simulink model "CANopen_CAN_Sender_Receiver"  (R2021b)
settings: Solver=VariableStepAuto  StartTime=0.0  StopTime=10.0  RelTol=1e-3
undefined symbols (not defined in the file): canChannel
libraries: simulink x48, commutil2 x5, canlib x3, dspindex x3, etargetslib x2, canmsglib x1
(part 1 of 2)
settings Model: Creator=adhip  LastModifiedBy=adhip

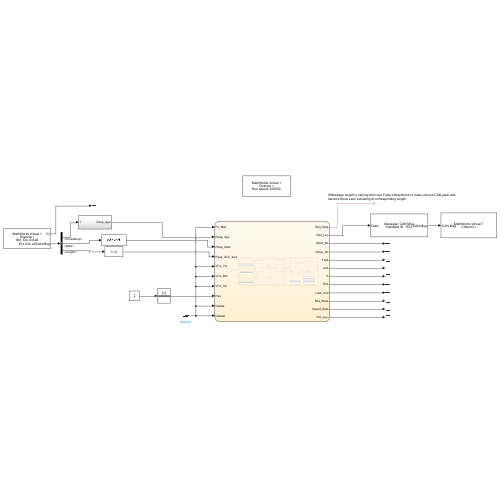
[thumbnail: Simulink's stored preview of the top-level diagram]
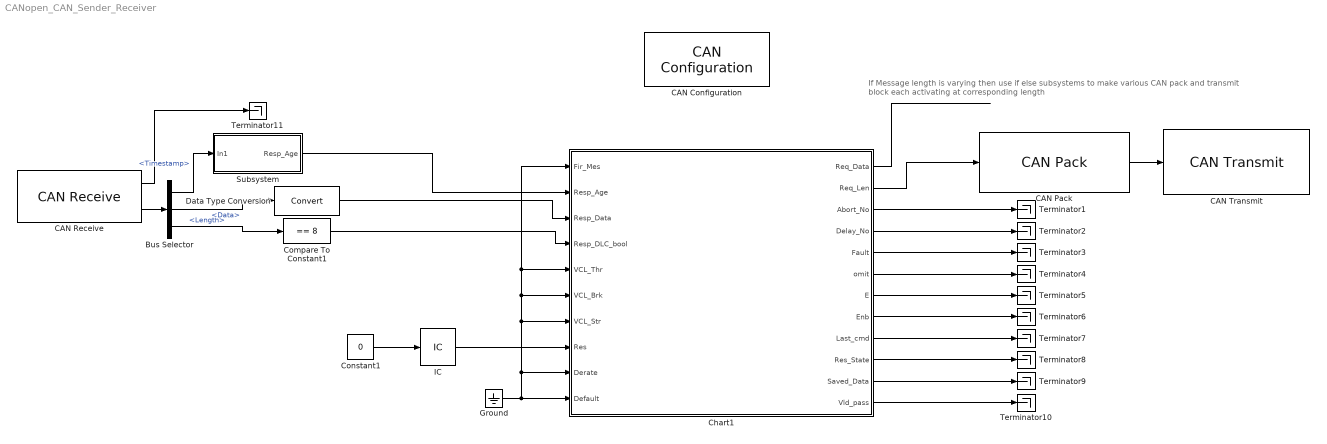
== system CANopen_CAN_Sender_Receiver ==
  note: If Message length is varying then use if else subsystems to make various CAN pack and transmit block each activating at corresponding length
  Bus Selector : BusSelector  OutputSignals=Timestamp,Data,Length
  CAN Configuration : canlib/CAN Configuration  BlockHandle=3200.0002  Device=MathWorks Virtual 1 (Channel 1)  DeviceMenu=MathWorks Virtual 1 (Channel 1)  ObjConstructor=canChannel('MathWorks', 'Virtual 1', 1)  BusSpeed=500000  EnableBitParameters=off  AckMode=Normal
      settings: SourceProductBaseCode=VN
  CAN Pack : canmsglib/CAN Pack  MsgList=(none)  MsgName=CAN Msg  MsgIDType=Standard (11-bit identifier)  MsgIdentifier=1574  MsgLength=8  Remote=off  ApplyMinMax=off  BusOutput=off  SignalInfo={}
      settings: SourceProductBaseCode=ME,XP,VN  DataFormat=raw data
  CAN Receive : canlib/CAN Receive  BlockHandle=3202.0002  Device=MathWorks Virtual 1 (Channel 1)  DeviceMenu=MathWorks Virtual 1 (Channel 1)  ObjConstructor=canChannel('MathWorks', 'Virtual 1', 1)  EnableStandardIDsFilter=off  StdIDsCombo=Allow only  StandardIDs=0x5a6  EnableExtendedIDsFilter=off  ExtIDsCombo=Allow all  ExtendedIDs=0  SampleTime=0.01  MsgsPerTimestep=all  InternalFilterUpdateStatus=on  BusOutput=on
      settings: SourceProductBaseCode=VN
  CAN Transmit : canlib/CAN Transmit  BlockHandle=3203.0002  Device=MathWorks Virtual 1 (Channel 1)  DeviceMenu=MathWorks Virtual 1 (Channel 1)  ObjConstructor=canChannel('MathWorks', 'Virtual 1', 1)  EnableEventTransmit=off  EnablePeriodicTransmit=off  MessagePeriod=1.000
      settings: SourceProductBaseCode=VN
  Chart1 : Stateflow chart  TreatAsAtomicUnit=on
      settings: PortSchema="{\"entries\":[{\"content\":{\"sides\":[{\"content\":{\"connectorIds\":[\"In10\",\"In1\",\"In3\",\"In2\",\"In4\",\"In5\",\"In6\",\"In9\",\"In7\",\"In8\"]},\"type\":\"ConnectorPlacement.EquallySpacedRectSide\",\"uuid\":\"d6208ab0-0bb6-4095-9d61-a018a45d5454\"},{\"content\":{\"connectorIds\":[\"Out1\",\"Out2\",\"Out3\",\"Out4\",\"Out5\",\"Out6\",\"Out7\",\"Out8\",\"Out9\",\"Out10\",\"Out11\",\"Out12\"],\"side\":\"RIGHT\"},\"type\":\"ConnectorPlacement.EquallySpacedRectSide\",\"uuid\":\"26e1aa46-d8b9-4154-9ae7-d888c7233d2e\"},{\"content\":{\"connectorIds\":[],\"side\":\"TOP\"},\"type\":\"ConnectorPlacement.EquallySpacedRectSide\",\"uuid\":\"42ea1899-a59d-4e0e-aa36-3438d8e67875\"}]},\"type\":\"ConnectorPlacement.EquallySpacedConnector\",\"uuid\":\"78564ca8-fcdf-4051-a3b6-ae8f3fd9c22a\"}],\"packageUris\":[\"http://schema.mathworks.com/mf0/Connector/R2020b\"],\"version\":\"1.0\"}"
  Compare To Constant1 : simulink/Logic and Bit Operations/Compare To Constant  relop===  const=8  OutDataTypeStr=boolean
  Constant1 : Constant  Value=0
  Data Type Conversion : DataTypeConversion
  Ground : Ground
  IC : InitialCondition
  Subsystem : Subsystem
  Terminator{1..11} (11 alike) : Terminator
  wires:
  Constant1/1 -> IC/1
  Ground/1 -> Chart1/8(Default), Chart1/6(VCL_Str), Chart1/5(VCL_Brk), Chart1/4(VCL_Thr), Chart1/10(Fir_Mes), Chart1/7(Derate)
  IC/1 -> Chart1/9(Res)
  CAN Receive/2 -> Bus Selector/1
  Bus Selector/3 -> Compare To Constant1/1  "<Length>"
  Compare To Constant1/1 -> Chart1/2(Resp_DLC_bool)
  Bus Selector/2 -> Data Type Conversion/1  "<Data>"
  Data Type Conversion/1 -> Chart1/3(Resp_Data)
  Bus Selector/1 -> Subsystem/1(In1)  "<Timestamp>"
  Subsystem/1(Resp_Age) -> Chart1/1(Resp_Age)
  Chart1/6(omit) -> Terminator4/1
  Chart1/11(Saved_Data) -> Terminator9/1
  Chart1/10(Res_State) -> Terminator8/1
  Chart1/7(E) -> Terminator5/1
  Chart1/9(Last_cmd) -> Terminator7/1
  Chart1/5(Fault) -> Terminator3/1
  Chart1/4(Delay_No) -> Terminator2/1
  Chart1/8(Enb) -> Terminator6/1
  Chart1/12(Vld_pass) -> Terminator10/1
  Chart1/3(Abort_No) -> Terminator1/1
  Chart1/1(Req_Data) -> ?
  CAN Pack/1 -> CAN Transmit/1
  Chart1/2(Req_Len) -> CAN Pack/1
  CAN Receive/1 -> Terminator11/1

== system CANopen_CAN_Sender_Receiver/Chart1/Transreceive.Identifying_Message.Disintegrate ==
  Data : Inport  OutDataTypeStr=uint8  PortDimensions=8
  f : TriggerPort  TriggerType=function-call  VariantControl=(inherit)
      settings: CopyFcn=Stateflow.SLINSF.SimulinkMan.removeBlockPreDeleteFcn  PreDeleteFcn=Stateflow.SLINSF.SimulinkMan.unsafePredeleteFcn
  Expedite : Subsystem
  Gains : Subsystem
  NOT : Logic  Operator=NOT  IconShape=distinctive  AllPortsSameDT=off  OutDataTypeStr=boolean
  Segmented : Subsystem  TreatAsAtomicUnit=on
  Subsystem : Subsystem
  Switch1 : Switch  Criteria=u2 > Threshold
  Switch2 : Switch  Criteria=u2 > Threshold
  Terminator : Terminator
  Terminator1 : Terminator
  Unit Delay : UnitDelay  SampleTime=-1  HasFrameUpgradeWarning=on
  Mes_No : Outport  OutDataTypeStr=uint8
  Act_Data : Outport  Port=2
  Seg_Req : Outport  Port=3  OutDataTypeStr=boolean
  Abort : Outport  Port=4  OutDataTypeStr=uint8
  wires:
  Switch1/1 -> Gains/2(Data)
  Data/1 -> Expedite/1(Data), Segmented/1(Data)
  Expedite/4("Request for Segmented Read ") -> Subsystem/1(set)
  Subsystem/1(Current State) -> Seg_Req/1, Unit Delay/1
  Segmented/1(Reset) -> Subsystem/2(Reset)
  NOT/1 -> Expedite/Enable, Switch2/2, Switch1/2
  Expedite/3(Act_Data) -> Switch1/1
  Expedite/2(Expedite) -> Terminator/1
  Segmented/2(Act_Data) -> Switch1/3
  Expedite/1(Msg No) -> Gains/1(Msg No), Mes_No/1
  Unit Delay/1 -> Segmented/Enable, NOT/1
  Expedite/5(Abort) -> Switch2/1
  Switch2/1 -> Abort/1
  Gains/1(Engineering value) -> Act_Data/1
  Segmented/4(Toggle) -> Terminator1/1
  Segmented/3(Abort) -> Switch2/3

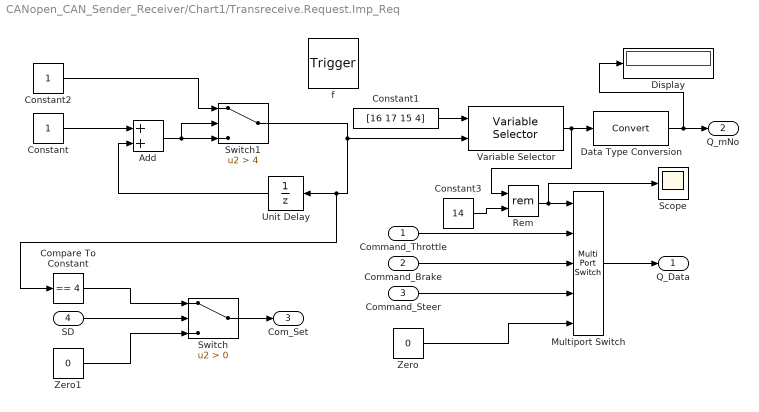
== system CANopen_CAN_Sender_Receiver/Chart1/Transreceive.Request.Imp_Req ==
  Command_Throttle : Inport  OutDataTypeStr=int8  PortDimensions=1
  Command_Brake : Inport  Port=2  OutDataTypeStr=int8  PortDimensions=1
  Command_Steer : Inport  Port=3  OutDataTypeStr=int8  PortDimensions=1
  SD : Inport  Port=4  OutDataTypeStr=boolean  PortDimensions=1
  f : TriggerPort  TriggerType=function-call  VariantControl=(inherit)
      settings: CopyFcn=Stateflow.SLINSF.SimulinkMan.removeBlockPreDeleteFcn  PreDeleteFcn=Stateflow.SLINSF.SimulinkMan.unsafePredeleteFcn
  Add : Sum
  Compare To Constant : simulink/Logic and Bit Operations/Compare To Constant  relop===  const=4  OutDataTypeStr=boolean
  Constant : Constant
  Constant1 : Constant  Value=[16 17 15 4]
  Constant2 : Constant
  Constant3 : Constant  Value=14
  Data Type Conversion : DataTypeConversion
  Display : Display
  Multiport Switch : MultiPortSwitch  Inputs=4  DiagnosticForDefault=None
  Rem : Math  Operator=rem  SaturateOnIntegerOverflow=on
  Scope : Scope
  Switch : Switch  Criteria=u2 > Threshold
  Switch1 : Switch  Criteria=u2 > Threshold  Threshold=4
  Unit Delay : UnitDelay  SampleTime=-1  HasFrameUpgradeWarning=on
  Variable Selector : dspindex/Variable Selector  NumInputs=1  rowsOrCols=Rows  IdxMode=Variable  Elements=[1 3]  ZerOneIdxMode=One-based  errmode=Clip Index  FillMode=on  FillValues=0
  Zero : Constant  Value=0  OutDataTypeStr=Inherit: Inherit via back propagation
  Zero1 : Constant  Value=0  OutDataTypeStr=Inherit: Inherit via back propagation
  Q_Data : Outport  OutDataTypeStr=uint16
  Q_mNo : Outport  Port=2  OutDataTypeStr=uint8
  Com_Set : Outport  Port=3
  wires:
  Unit Delay/1 -> Add/2
  Add/1 -> Switch1/2, Switch1/3
  Multiport Switch/1 -> Q_Data/1
  Command_Steer/1 -> Multiport Switch/4
  Command_Brake/1 -> Multiport Switch/3
  Command_Throttle/1 -> Multiport Switch/2
  Constant3/1 -> Rem/2
  Constant1/1 -> Variable Selector/1
  Constant/1 -> Add/1
  Variable Selector/1 -> Rem/1, Data Type Conversion/1
  Constant2/1 -> Switch1/1
  Zero/1 -> Multiport Switch/5
  Switch1/1 -> Compare To Constant/1, Unit Delay/1, Variable Selector/2
  Rem/1 -> Scope/1, Multiport Switch/1
  Compare To Constant/1 -> Switch/1
  Switch/1 -> Com_Set/1
  SD/1 -> Switch/2
  Zero1/1 -> Switch/3
  Data Type Conversion/1 -> Q_mNo/1, Display/1

== system CANopen_CAN_Sender_Receiver/Chart1/Transreceive.Request.Logic_Based ==
  f : TriggerPort  TriggerType=function-call  VariantControl=(inherit)
      settings: CopyFcn=Stateflow.SLINSF.SimulinkMan.removeBlockPreDeleteFcn  PreDeleteFcn=Stateflow.SLINSF.SimulinkMan.unsafePredeleteFcn
  Add : Sum
  Constant : Constant
  Constant1 : Constant  Value=[12 13 10 11]
  Constant2 : Constant
  Data Type Conversion : DataTypeConversion
  Display : Display
  Switch1 : Switch  Criteria=u2 > Threshold  Threshold=4
  Unit Delay : UnitDelay  SampleTime=-1  HasFrameUpgradeWarning=on
  Variable Selector : dspindex/Variable Selector  NumInputs=1  rowsOrCols=Rows  IdxMode=Variable  Elements=[1 3]  ZerOneIdxMode=One-based  errmode=Clip Index  FillMode=on  FillValues=0
  Zero : Constant  Value=0  OutDataTypeStr=Inherit: Inherit via back propagation
  Zero1 : Constant  Value=0  OutDataTypeStr=Inherit: Inherit via back propagation
  Q_Data : Outport  OutDataTypeStr=uint16
  Q_mNo : Outport  Port=2  OutDataTypeStr=uint8
  Com_Set : Outport  Port=3
  wires:
  Unit Delay/1 -> Add/2
  Add/1 -> Switch1/2, Switch1/3
  Constant1/1 -> Variable Selector/1
  Constant/1 -> Add/1
  Variable Selector/1 -> Data Type Conversion/1
  Constant2/1 -> Switch1/1
  Zero/1 -> Q_Data/1
  Switch1/1 -> Variable Selector/2, Unit Delay/1
  Zero1/1 -> Com_Set/1
  Data Type Conversion/1 -> Q_mNo/1, Display/1

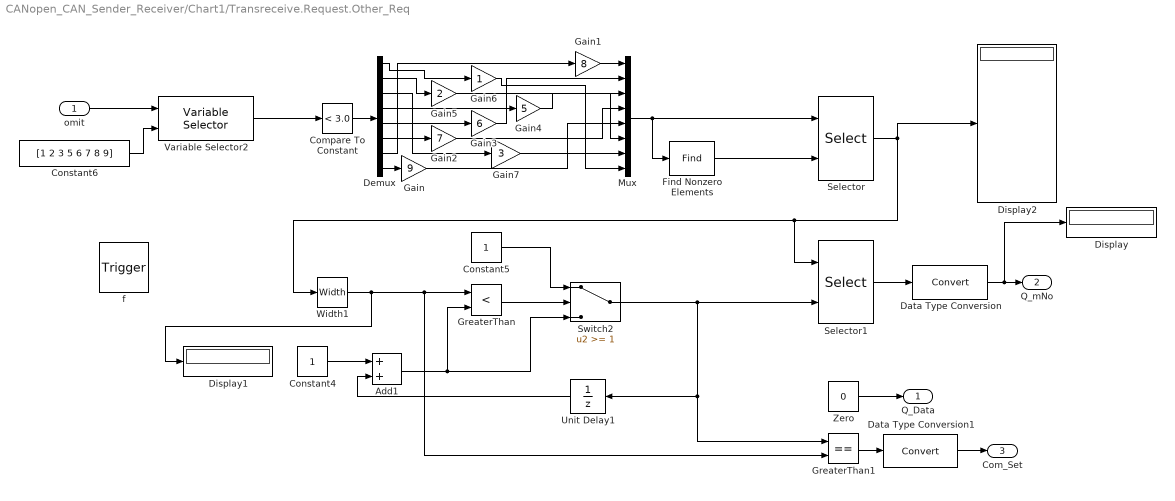
== system CANopen_CAN_Sender_Receiver/Chart1/Transreceive.Request.Other_Req ==
  omit : Inport  OutDataTypeStr=uint8  PortDimensions=17
  f : TriggerPort  TriggerType=function-call  VariantControl=(inherit)
      settings: CopyFcn=Stateflow.SLINSF.SimulinkMan.removeBlockPreDeleteFcn  PreDeleteFcn=Stateflow.SLINSF.SimulinkMan.unsafePredeleteFcn
  Add1 : Sum
  Compare To Constant : simulink/Logic and Bit Operations/Compare To Constant  relop=<  const=3.0  OutDataTypeStr=boolean
  Constant4 : Constant
  Constant5 : Constant
  Constant6 : Constant  Value=[1 2 3 5 6 7 8 9]
  Data Type Conversion : DataTypeConversion
  Data Type Conversion1 : DataTypeConversion
  Demux : Demux  Outputs=8
  Display : Display
  Display1 : Display
  Display2 : Display
  Find Nonzero Elements : Find  NumberOfInputDimensions=3
  Gain : Gain  Gain=9  OutDataTypeStr=uint8
  Gain1 : Gain  Gain=8  OutDataTypeStr=uint8
  Gain2 : Gain  Gain=7  OutDataTypeStr=uint8
  Gain3 : Gain  Gain=6  OutDataTypeStr=uint8
  Gain4 : Gain  Gain=5  OutDataTypeStr=uint8
  Gain5 : Gain  Gain=2  OutDataTypeStr=uint8
  Gain6 : Gain  OutDataTypeStr=uint8
  Gain7 : Gain  Gain=3  OutDataTypeStr=uint8
  GreaterThan : RelationalOperator  Operator=<  OutDataTypeStr=boolean  RndMeth=Simplest
  GreaterThan1 : RelationalOperator  Operator===  OutDataTypeStr=boolean  RndMeth=Simplest
  Mux : Mux  Inputs=8
  Selector : Selector  InputPortWidth=8  IndexOptions=Index vector (port)  Indices=[1 3]  OutputSizes=1
  Selector1 : Selector  InputPortWidth=8  IndexOptions=Index vector (port)  Indices=[1 3]  OutputSizes=1
  Switch2 : Switch  Threshold=1
  Unit Delay1 : UnitDelay  SampleTime=-1  HasFrameUpgradeWarning=on
  Variable Selector2 : dspindex/Variable Selector  NumInputs=1  rowsOrCols=Rows  IdxMode=Variable  Elements=[1 3]  ZerOneIdxMode=One-based  errmode=Clip Index  FillMode=on  FillValues=0
  Width1 : Width
  Zero : Constant  Value=0  OutDataTypeStr=Inherit: Inherit via back propagation
  Q_Data : Outport  OutDataTypeStr=uint16
  Q_mNo : Outport  Port=2  OutDataTypeStr=uint8
  Com_Set : Outport  Port=3
  wires:
  Zero/1 -> Q_Data/1
  Switch2/1 -> Selector1/2, GreaterThan1/1, Unit Delay1/1
  Gain/1 -> Mux/5
  Gain6/1 -> Mux/8
  Demux/7 -> Gain1/1
  Demux/1 -> Gain6/1
  Gain3/1 -> Mux/2
  Gain5/1 -> Mux/6
  Demux/3 -> Gain7/1
  Demux/4 -> Gain4/1
  Demux/2 -> Gain5/1
  Mux/1 -> Selector/1, Find Nonzero Elements/1
  Demux/8 -> Gain/1
  Width1/1 -> GreaterThan1/2, GreaterThan/1, Display1/1
  Constant6/1 -> Variable Selector2/2
  Compare To Constant/1 -> Demux/1
  Demux/6 -> Gain2/1
  Constant5/1 -> Switch2/1
  Unit Delay1/1 -> Add1/2
  Demux/5 -> Gain3/1
  Gain4/1 -> Mux/3
  Constant4/1 -> Add1/1
  Add1/1 -> GreaterThan/2, Switch2/3
  Gain2/1 -> Mux/4
  Selector1/1 -> Data Type Conversion/1
  Selector/1 -> Selector1/1, Width1/1, Display2/1
  Variable Selector2/1 -> Compare To Constant/1
  GreaterThan/1 -> Switch2/2
  omit/1 -> Variable Selector2/1
  Gain7/1 -> Mux/7
  Find Nonzero Elements/1 -> Selector/2
  Gain1/1 -> Mux/1
  GreaterThan1/1 -> Data Type Conversion1/1
  Data Type Conversion/1 -> Q_mNo/1, Display/1
  Data Type Conversion1/1 -> Com_Set/1

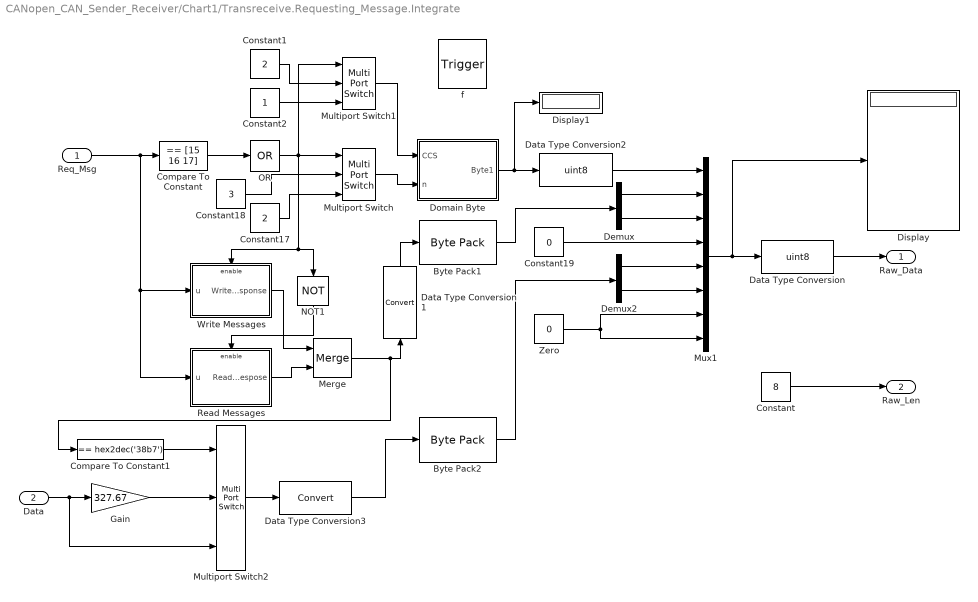
== system CANopen_CAN_Sender_Receiver/Chart1/Transreceive.Requesting_Message.Integrate ==
  Req_Msg : Inport  OutDataTypeStr=uint8  PortDimensions=1
  Data : Inport  Port=2  OutDataTypeStr=uint16  PortDimensions=1
  f : TriggerPort  TriggerType=function-call  VariantControl=(inherit)
      settings: CopyFcn=Stateflow.SLINSF.SimulinkMan.removeBlockPreDeleteFcn  PreDeleteFcn=Stateflow.SLINSF.SimulinkMan.unsafePredeleteFcn
  Byte Pack1 : etargetslib/Byte Pack  datatypes={'uint16'}  byteAlign=1
  Byte Pack2 : etargetslib/Byte Pack  datatypes={'uint16'}  byteAlign=1
  Compare To Constant : simulink/Logic and Bit Operations/Compare To Constant  relop===  const=[15 16 17]  OutDataTypeStr=boolean
  Compare To Constant1 : simulink/Logic and Bit Operations/Compare To Constant  relop===  const=hex2dec('38b7')  OutDataTypeStr=boolean
  Constant : Constant  Value=8  OutDataTypeStr=uint8
  Constant1 : Constant  Value=2
  Constant17 : Constant  Value=2
  Constant18 : Constant  Value=3
  Constant19 : Constant  Value=0  OutDataTypeStr=uint8
  Constant2 : Constant
  Data Type Conversion : DataTypeConversion  OutDataTypeStr=uint8
  Data Type Conversion1 : DataTypeConversion
  Data Type Conversion2 : DataTypeConversion  OutDataTypeStr=uint8
  Data Type Conversion3 : DataTypeConversion
  Demux : Demux  Outputs=2
  Demux2 : Demux  Outputs=2
  Display : Display
  Display1 : Display
  Domain Byte : Subsystem
  Gain : Gain  Gain=327.67
  Merge : Merge
  Multiport Switch : MultiPortSwitch  DataPortOrder=Zero-based contiguous  Inputs=2  zeroidx=on
  Multiport Switch1 : MultiPortSwitch  DataPortOrder=Zero-based contiguous  Inputs=2  zeroidx=on
  Multiport Switch2 : MultiPortSwitch  DataPortOrder=Zero-based contiguous  Inputs=2  zeroidx=on
  Mux1 : Mux  Inputs=8
  NOT1 : Logic  Operator=NOT  IconShape=distinctive  AllPortsSameDT=off  OutDataTypeStr=boolean
  OR : Logic  Operator=OR  Inputs=1  IconShape=distinctive  AllPortsSameDT=off  OutDataTypeStr=boolean
  Read Messages : Subsystem
  Write Messages : Subsystem
  Zero : Constant  Value=0  OutDataTypeStr=uint8
  Raw_Data : Outport
  Raw_Len : Outport  Port=2
  wires:
  Gain/1 -> Multiport Switch2/2
  Compare To Constant1/1 -> Multiport Switch2/1
  Data Type Conversion3/1 -> Byte Pack2/1
  Multiport Switch2/1 -> Data Type Conversion3/1
  Multiport Switch1/1 -> Domain Byte/1(CCS)
  Constant2/1 -> Multiport Switch1/3
  Constant1/1 -> Multiport Switch1/2
  Data Type Conversion1/1 -> Byte Pack1/1
  Demux/1 -> Mux1/2
  Data Type Conversion2/1 -> Mux1/1
  Demux2/1 -> Mux1/5
  Demux/2 -> Mux1/3
  Data/1 -> Gain/1, Multiport Switch2/3
  Byte Pack1/1 -> Demux/1
  Byte Pack2/1 -> Demux2/1
  Domain Byte/1(Byte1) -> Data Type Conversion2/1, Display1/1
  Constant19/1 -> Mux1/4
  NOT1/1 -> Read Messages/Enable
  Read Messages/1(Read_Respose) -> Merge/2
  Mux1/1 -> Data Type Conversion/1, Display/1
  Zero/1 -> Mux1/8, Mux1/7
  OR/1 -> Write Messages/Enable, NOT1/1, Multiport Switch/1, Multiport Switch1/1
  Constant18/1 -> Multiport Switch/2
  Compare To Constant/1 -> OR/1
  Demux2/2 -> Mux1/6
  Req_Msg/1 -> Read Messages/1(u), Write Messages/1(u), Compare To Constant/1
  Constant17/1 -> Multiport Switch/3
  Data Type Conversion/1 -> Raw_Data/1
  Write Messages/1(Write_response) -> Merge/1
  Merge/1 -> Data Type Conversion1/1, Compare To Constant1/1
  Multiport Switch/1 -> Domain Byte/2(n)
  Constant/1 -> Raw_Len/1

== system CANopen_CAN_Sender_Receiver/Subsystem ==
  note: Create a system that comapres time stamp with atcual time and gives age 0 if a fresh message is received
  In1 : Inport
  Clock : Clock
  Resp_Age : Outport

== system CANopen_CAN_Sender_Receiver/Chart1/Transreceive.Identifying_Message.Disintegrate/Expedite ==
  Data : Inport
  Enable : EnablePort
  Data Processing : Subsystem
  Demux : Demux  Outputs=8
  Display{,1..3} (4 alike) : Display
  MessageNumber : Subsystem
  Mux : Mux  Inputs=3
  Mux1 : Mux
  Msg No : Outport
  Expedite : Outport  Port=2
  Act_Data : Outport  Port=3
  "Request for Segmented Read " : Outport  Port=4
  Abort : Outport  Port=5
  wires:
  Demux/8 -> Mux1/4
  Demux/3 -> Mux/2
  Demux/5 -> Mux1/1
  Demux/7 -> Mux1/3
  Mux/1 -> MessageNumber/2(u)
  Demux/4 -> Mux/3
  Demux/2 -> Mux/1
  Mux1/1 -> Data Processing/2(In1), Display/1
  Demux/6 -> Mux1/2
  Demux/1 -> MessageNumber/1(Domain Info)
  MessageNumber/1(Msg No) -> Data Processing/1(Msg No), Msg No/1, Display1/1
  MessageNumber/2(Expedite) -> Expedite/1
  Data/1 -> Demux/1, Display2/1
  MessageNumber/3("Request for Segmented Read ") -> "Request for Segmented Read "/1
  Data Processing/1(Act_Data) -> Act_Data/1, Display3/1
  MessageNumber/4(Abort) -> Abort/1

== system CANopen_CAN_Sender_Receiver/Chart1/Transreceive.Identifying_Message.Disintegrate/Gains ==
  Msg No : Inport
  Data : Inport  Port=2
  Constant : Constant  Value=[327.67, 327.67, 1, 1, 10, 10, 10, 1, 1, 40.96, 40.96, 40.96, 40.96, 105, 1, 1, 1, 1]
  Demux : Demux  Outputs=18
  Display : Display
  Display1 : Display
  Divide : Product  Inputs=*/
  Multiport Switch : MultiPortSwitch  Inputs=18
  Engineering value : Outport
  wires:
  Multiport Switch/1 -> Divide/2, Display/1
  Data/1 -> Divide/1
  Divide/1 -> Engineering value/1, Display1/1
  Msg No/1 -> Multiport Switch/1
  Demux/1 -> Multiport Switch/2
  Demux/2 -> Multiport Switch/3
  Demux/3 -> Multiport Switch/4
  Demux/4 -> Multiport Switch/5
  Demux/5 -> Multiport Switch/6
  Demux/6 -> Multiport Switch/7
  Demux/7 -> Multiport Switch/8
  Demux/8 -> Multiport Switch/9
  Demux/9 -> Multiport Switch/10
  Demux/10 -> Multiport Switch/11
  Demux/11 -> Multiport Switch/12
  Demux/12 -> Multiport Switch/13
  Demux/13 -> Multiport Switch/14
  Demux/14 -> Multiport Switch/15
  Demux/15 -> Multiport Switch/16
  Demux/16 -> Multiport Switch/17
  Demux/17 -> Multiport Switch/18
  Demux/18 -> Multiport Switch/19
  Constant/1 -> Demux/1

== system CANopen_CAN_Sender_Receiver/Chart1/Transreceive.Identifying_Message.Disintegrate/Segmented ==
  Data : Inport
  Enable : EnablePort
  Data Processing : Subsystem
  Demux : Demux  Outputs=8
  MessageNumber : Subsystem
  Mux1 : Mux  Inputs=7
  Terminator : Terminator
  Terminator1 : Terminator
  Reset : Outport
  Act_Data : Outport  Port=2
  Abort : Outport  Port=3
  Toggle : Outport  Port=4
  wires:
  Demux/1 -> MessageNumber/1(Domain Info)
  Data/1 -> Demux/1
  Mux1/1 -> Data Processing/1(Data)
  Demux/2 -> Mux1/1
  Demux/4 -> Mux1/3
  Demux/3 -> Mux1/2
  MessageNumber/2(Reset) -> Reset/1
  Demux/5 -> Mux1/4
  Demux/6 -> Mux1/5
  Demux/7 -> Mux1/6
  Demux/8 -> Mux1/7
  Data Processing/1(Act_Data) -> Act_Data/1
  MessageNumber/1(Abort) -> Abort/1
  MessageNumber/3(Toggle) -> Toggle/1
  MessageNumber/5(Segmented Response) -> Terminator/1
  MessageNumber/4(Error SCS) -> Terminator1/1

== system CANopen_CAN_Sender_Receiver/Chart1/Transreceive.Identifying_Message.Disintegrate/Subsystem ==
  set : Inport
  Reset : Inport  Port=2
  Constant : Constant  Value=0  OutDataTypeStr=boolean
  Constant1 : Constant  OutDataTypeStr=boolean
  Multiport Switch : MultiPortSwitch  DataPortOrder=Zero-based contiguous  Inputs=2  zeroidx=on
  Multiport Switch1 : MultiPortSwitch  DataPortOrder=Zero-based contiguous  Inputs=2  zeroidx=on
  Unit Delay : UnitDelay  SampleTime=-1  HasFrameUpgradeWarning=on
  Current State : Outport
  wires:
  Multiport Switch/1 -> Current State/1, Unit Delay/1
  Constant/1 -> Multiport Switch/3
  Multiport Switch1/1 -> Multiport Switch/2
  Constant1/1 -> Multiport Switch1/3
  Unit Delay/1 -> Multiport Switch1/2
  Reset/1 -> Multiport Switch/1
  set/1 -> Multiport Switch1/1

== system CANopen_CAN_Sender_Receiver/Chart1/Transreceive.Requesting_Message.Integrate/Domain Byte ==
  CCS : Inport
  n : Inport  Port=2
  Bit to Integer Converter : commutil2/Bit to Integer Converter  nbits=8  bitOrder=MSB first  signedOutputValues=Unsigned  outDtype=Inherit via internal rule  outDtypeSigned=Inherit via internal rule
      settings: SourceProductBaseCode=SL
  Constant : Constant  Value=0
  Constant1 : Constant  Value=0
  Constant2 : Constant
  Constant3 : Constant  Value=0
  Constant4 : Constant
  Constant5 : Constant
  Demux : Demux  Outputs=2
  Demux1 : Demux  Outputs=2
  Display1 : Display
  Display2 : Display
  Integer to Bit Converter : commutil2/Integer to Bit Converter  nbits=2  signedInputValues=Unsigned  bitOrder=MSB first  outDtype=Inherit via internal rule
      settings: SourceProductBaseCode=SL
  Integer to Bit Converter1 : commutil2/Integer to Bit Converter  nbits=2  signedInputValues=Unsigned  bitOrder=MSB first  outDtype=Inherit via internal rule
      settings: SourceProductBaseCode=SL
  Mux : Mux  Inputs=8
  Byte1 : Outport
  wires:
  CCS/1 -> Integer to Bit Converter1/1
  Integer to Bit Converter1/1 -> Demux1/1, Display2/1
  Mux/1 -> Bit to Integer Converter/1, Display1/1
  Bit to Integer Converter/1 -> Byte1/1
  Demux1/1 -> Mux/2
  Demux1/2 -> Mux/3
  Constant4/1 -> Mux/8
  Constant/1 -> Mux/1
  Constant3/1 -> Mux/4
  Constant5/1 -> Mux/7
  n/1 -> Integer to Bit Converter/1
  Integer to Bit Converter/1 -> Demux/1
  Demux/1 -> Mux/5
  Demux/2 -> Mux/6

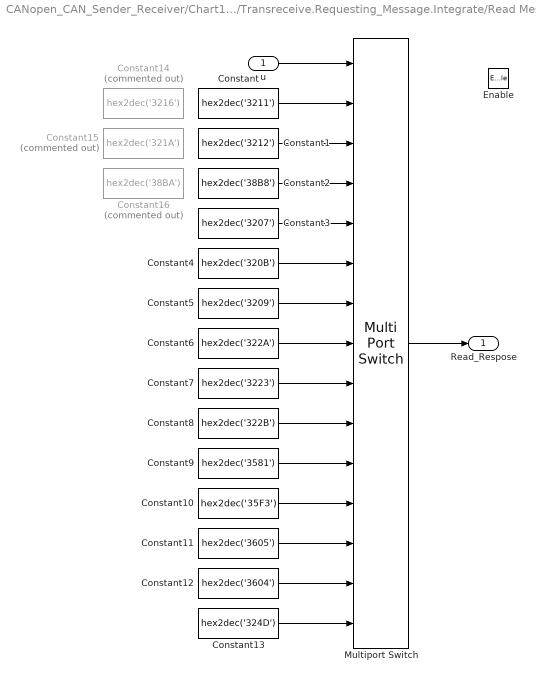
== system CANopen_CAN_Sender_Receiver/Chart1/Transreceive.Requesting_Message.Integrate/Read Messages ==
  u : Inport
  Enable : EnablePort  StatesWhenEnabling=reset
  Constant : Constant  Value=hex2dec('3211')
  Constant1 : Constant  Value=hex2dec('3212')
  Constant10 : Constant  Value=hex2dec('35F3')
  Constant11 : Constant  Value=hex2dec('3605')
  Constant12 : Constant  Value=hex2dec('3604')
  Constant13 : Constant  Value=hex2dec('324D')
  Constant14 : Constant  Commented=on  Value=hex2dec('3216')
  Constant15 : Constant  Commented=on  Value=hex2dec('321A')
  Constant16 : Constant  Commented=on  Value=hex2dec('38BA')
  Constant2 : Constant  Value=hex2dec('38B8')
  Constant3 : Constant  Value=hex2dec('3207')
  Constant4 : Constant  Value=hex2dec('320B')
  Constant5 : Constant  Value=hex2dec('3209')
  Constant6 : Constant  Value=hex2dec('322A')
  Constant7 : Constant  Value=hex2dec('3223')
  Constant8 : Constant  Value=hex2dec('322B')
  Constant9 : Constant  Value=hex2dec('3581')
  Multiport Switch : MultiPortSwitch  Inputs=14
  Read_Respose : Outport
  wires:
  u/1 -> Multiport Switch/1
  Constant/1 -> Multiport Switch/2
  Constant1/1 -> Multiport Switch/3
  Constant3/1 -> Multiport Switch/5
  Constant2/1 -> Multiport Switch/4
  Constant7/1 -> Multiport Switch/9
  Constant6/1 -> Multiport Switch/8
  Constant5/1 -> Multiport Switch/7
  Constant4/1 -> Multiport Switch/6
  Constant8/1 -> Multiport Switch/10
  Constant9/1 -> Multiport Switch/11
  Constant10/1 -> Multiport Switch/12
  Constant11/1 -> Multiport Switch/13
  Constant12/1 -> Multiport Switch/14
  Constant13/1 -> Multiport Switch/15
  Multiport Switch/1 -> Read_Respose/1

== system CANopen_CAN_Sender_Receiver/Chart1/Transreceive.Requesting_Message.Integrate/Write Messages ==
  u : Inport
  Enable : EnablePort  StatesWhenEnabling=reset
  Add : Sum  Inputs=+++
  Constant : Constant  Value=hex2dec('3218')
  Constant1 : Constant  Value=hex2dec('3219')
  Constant2 : Constant  Value=hex2dec('38b7')
  Gain1 : Gain  Gain=2  OutDataTypeStr=uint16
  Gain3 : Gain  Gain=3  OutDataTypeStr=uint16
  Multiport Switch : MultiPortSwitch
  VCL_Brake : simulink/Logic and Bit Operations/Compare To Constant  relop===  const=16  OutDataTypeStr=uint8
  VCL_Steer : simulink/Logic and Bit Operations/Compare To Constant  relop===  const=17  OutDataTypeStr=uint8
  VCL_Throttle : simulink/Logic and Bit Operations/Compare To Constant  relop===  const=15  OutDataTypeStr=uint8
  Write_response : Outport
  wires:
  VCL_Brake/1 -> Gain1/1
  u/1 -> VCL_Steer/1, VCL_Brake/1, VCL_Throttle/1
  VCL_Steer/1 -> Gain3/1
  Multiport Switch/1 -> Write_response/1
  Gain1/1 -> Add/2
  VCL_Throttle/1 -> Add/1
  Gain3/1 -> Add/3
  Add/1 -> Multiport Switch/1
  Constant/1 -> Multiport Switch/2
  Constant2/1 -> Multiport Switch/4
  Constant1/1 -> Multiport Switch/3

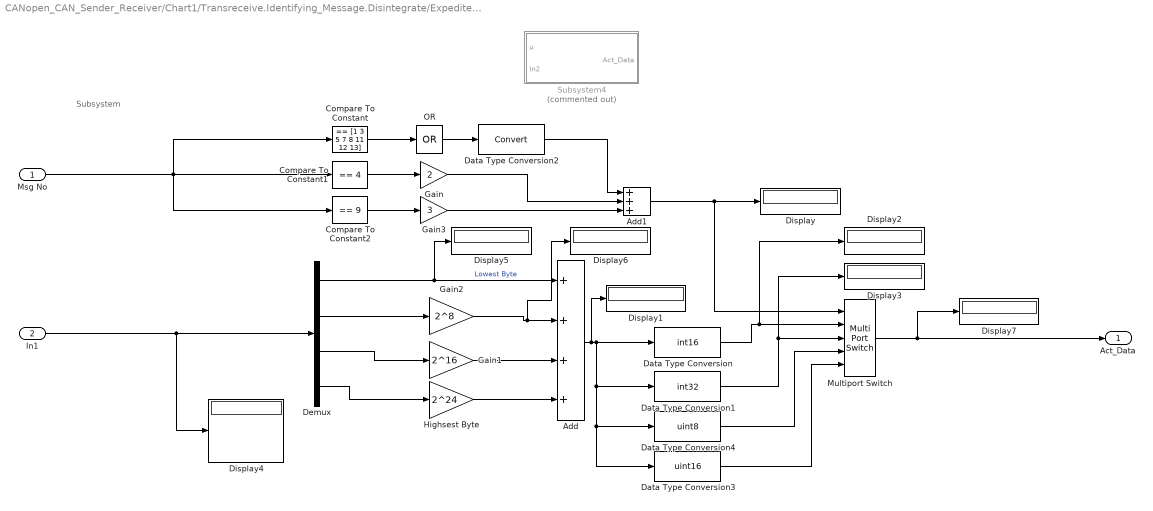
== system CANopen_CAN_Sender_Receiver/Chart1/Transreceive.Identifying_Message.Disintegrate/Expedite/Data Processing ==
  note: Subsystem
  Msg No : Inport
  In1 : Inport  Port=2
  Add : Sum  Inputs=++++  OutDataTypeStr=uint32
  Add1 : Sum  Inputs=+++
  Compare To Constant : simulink/Logic and Bit Operations/Compare To Constant  relop===  const=[1 3 5 7 8 11 12 13]  OutDataTypeStr=boolean
  Compare To Constant1 : simulink/Logic and Bit Operations/Compare To Constant  relop===  const=4  OutDataTypeStr=boolean
  Compare To Constant2 : simulink/Logic and Bit Operations/Compare To Constant  relop===  const=9  OutDataTypeStr=boolean
  Data Type Conversion : DataTypeConversion  OutDataTypeStr=int16  SaturateOnIntegerOverflow=on
  Data Type Conversion1 : DataTypeConversion  OutDataTypeStr=int32  SaturateOnIntegerOverflow=on
  Data Type Conversion2 : DataTypeConversion
  Data Type Conversion3 : DataTypeConversion  OutDataTypeStr=uint16  SaturateOnIntegerOverflow=on
  Data Type Conversion4 : DataTypeConversion  OutDataTypeStr=uint8  SaturateOnIntegerOverflow=on
  Demux : Demux
  Display{,1..7} (8 alike) : Display
  Gain : Gain  Gain=2
  Gain1 : Gain  Gain=2^16
  Gain2 : Gain  Gain=2^8
  Gain3 : Gain  Gain=3
  Highsest Byte : Gain  Gain=2^24
  Multiport Switch : MultiPortSwitch  Inputs=4  DiagnosticForDefault=None  OutDataTypeStr=double
  OR : Logic  Operator=OR  Inputs=1  IconShape=distinctive  AllPortsSameDT=off  OutDataTypeStr=boolean
  Subsystem4 : Subsystem  Commented=on
  Act_Data : Outport
  wires:
  Gain/1 -> Add1/2
  In1/1 -> Display4/1, Demux/1
  Demux/4 -> Highsest Byte/1
  Add1/1 -> Multiport Switch/1, Display/1
  Data Type Conversion4/1 -> Multiport Switch/4
  Data Type Conversion1/1 -> Multiport Switch/3, Display3/1
  Data Type Conversion2/1 -> Add1/1
  Compare To Constant/1 -> OR/1
  Compare To Constant2/1 -> Gain3/1
  Gain3/1 -> Add1/3
  Highsest Byte/1 -> Add/4
  OR/1 -> Data Type Conversion2/1
  Demux/1 -> Display5/1, Add/1  "Lowest Byte"
  Data Type Conversion3/1 -> Multiport Switch/5
  Gain2/1 -> Display6/1, Add/2
  Gain1/1 -> Add/3
  Data Type Conversion/1 -> Multiport Switch/2, Display2/1
  Compare To Constant1/1 -> Gain/1
  Demux/2 -> Gain2/1
  Demux/3 -> Gain1/1
  Msg No/1 -> Compare To Constant/1, Compare To Constant1/1, Compare To Constant2/1
  Add/1 -> Display1/1, Data Type Conversion/1, Data Type Conversion1/1, Data Type Conversion4/1, Data Type Conversion3/1
  Multiport Switch/1 -> Display7/1, Act_Data/1

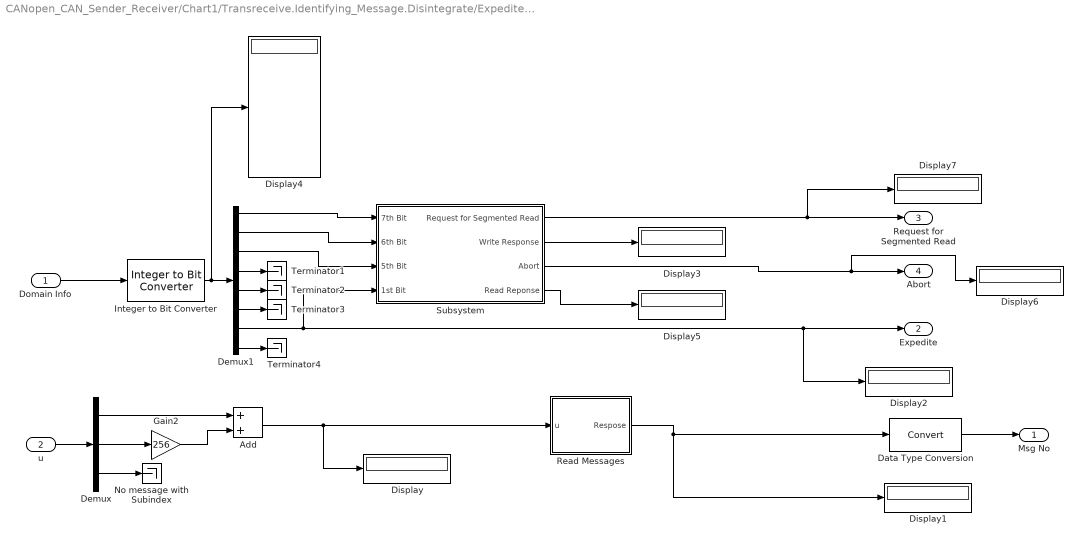
== system CANopen_CAN_Sender_Receiver/Chart1/Transreceive.Identifying_Message.Disintegrate/Expedite/MessageNumber ==
  Domain Info : Inport
  u : Inport  Port=2
  Add : Sum  OutDataTypeStr=uint16
  Data Type Conversion : DataTypeConversion
  Demux : Demux  Outputs=3
  Demux1 : Demux  Outputs=8
  Display{,1..7} (8 alike) : Display
  Gain2 : Gain  Gain=256
  Integer to Bit Converter : commutil2/Integer to Bit Converter  nbits=8  signedInputValues=Unsigned  bitOrder=MSB first  outDtype=Inherit via internal rule
      settings: SourceProductBaseCode=SL
  No message with Subindex : Terminator
  Read Messages : Subsystem
  Subsystem : Subsystem
  Terminator{1..4} (4 alike) : Terminator
  Msg No : Outport
  Expedite : Outport  Port=2
  "Request for Segmented Read " : Outport  Port=3
  Abort : Outport  Port=4
  wires:
  Subsystem/2(Write Response) -> Display3/1
  Data Type Conversion/1 -> Msg No/1
  Read Messages/1(Respose) -> Display1/1, Data Type Conversion/1
  u/1 -> Demux/1
  Demux/2 -> Gain2/1
  Demux/1 -> Add/1
  Gain2/1 -> Add/2
  Add/1 -> Read Messages/1(u), Display/1
  Demux/3 -> No message with Subindex/1
  Domain Info/1 -> Integer to Bit Converter/1
  Integer to Bit Converter/1 -> Demux1/1, Display4/1
  Demux1/7 -> Expedite/1, Display2/1, Subsystem/4(1st Bit)
  Demux1/4 -> Terminator1/1
  Demux1/5 -> Terminator2/1
  Demux1/6 -> Terminator3/1
  Demux1/8 -> Terminator4/1
  Demux1/1 -> Subsystem/1(7th Bit)
  Demux1/2 -> Subsystem/2(6th Bit)
  Demux1/3 -> Subsystem/3(5th Bit)
  Subsystem/4(Read Reponse) -> Display5/1
  Subsystem/1("Request for Segmented Read ") -> "Request for Segmented Read "/1, Display7/1
  Subsystem/3(Abort) -> Abort/1, Display6/1

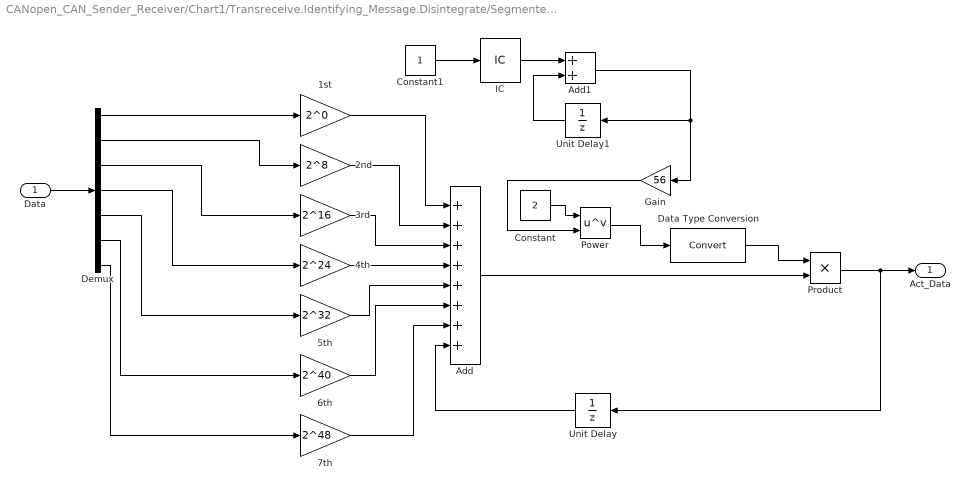
== system CANopen_CAN_Sender_Receiver/Chart1/Transreceive.Identifying_Message.Disintegrate/Segmented/Data Processing ==
  Data : Inport
  1st : Gain  Gain=2^0
  2nd : Gain  Gain=2^8
  3rd : Gain  Gain=2^16
  4th : Gain  Gain=2^24
  5th : Gain  Gain=2^32
  6th : Gain  Gain=2^40
  7th : Gain  Gain=2^48
  Add : Sum  Inputs=++++++++
  Add1 : Sum
  Constant : Constant  Value=2
  Constant1 : Constant
  Data Type Conversion : DataTypeConversion
  Demux : Demux  Outputs=7
  Gain : Gain  Gain=56
  IC : InitialCondition  Value=0
  Power : Math  Operator=pow  SaturateOnIntegerOverflow=on
  Product : Product  OutDataTypeStr=double
  Unit Delay : UnitDelay  SampleTime=-1  HasFrameUpgradeWarning=on
  Unit Delay1 : UnitDelay  SampleTime=-1  HasFrameUpgradeWarning=on
  Act_Data : Outport
  wires:
  Data/1 -> Demux/1
  Demux/4 -> 4th/1
  Demux/3 -> 3rd/1
  Demux/2 -> 2nd/1
  4th/1 -> Add/4
  3rd/1 -> Add/3
  2nd/1 -> Add/2
  Demux/1 -> 1st/1
  Product/1 -> Unit Delay/1, Act_Data/1
  Demux/5 -> 5th/1
  Demux/6 -> 6th/1
  Demux/7 -> 7th/1
  5th/1 -> Add/5
  6th/1 -> Add/6
  7th/1 -> Add/7
  Unit Delay/1 -> Add/8
  1st/1 -> Add/1
  Add/1 -> Product/2
  Constant/1 -> Power/1
  Power/1 -> Data Type Conversion/1
  Constant1/1 -> IC/1
  Add1/1 -> Gain/1, Unit Delay1/1
  Unit Delay1/1 -> Add1/2
  IC/1 -> Add1/1
  Gain/1 -> Power/2
  Data Type Conversion/1 -> Product/1

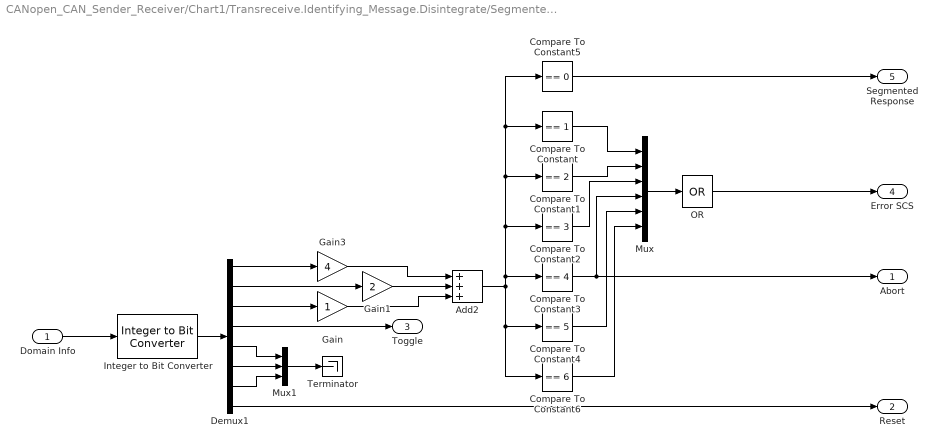
== system CANopen_CAN_Sender_Receiver/Chart1/Transreceive.Identifying_Message.Disintegrate/Segmented/MessageNumber ==
  Domain Info : Inport
  Add2 : Sum  Inputs=+++
  Compare To Constant : simulink/Logic and Bit Operations/Compare To Constant  relop===  const=1  OutDataTypeStr=boolean
  Compare To Constant1 : simulink/Logic and Bit Operations/Compare To Constant  relop===  const=2  OutDataTypeStr=boolean
  Compare To Constant2 : simulink/Logic and Bit Operations/Compare To Constant  relop===  const=3  OutDataTypeStr=boolean
  Compare To Constant3 : simulink/Logic and Bit Operations/Compare To Constant  relop===  const=4  OutDataTypeStr=boolean
  Compare To Constant4 : simulink/Logic and Bit Operations/Compare To Constant  relop===  const=5  OutDataTypeStr=boolean
  Compare To Constant5 : simulink/Logic and Bit Operations/Compare To Constant  relop===  const=0  OutDataTypeStr=boolean
  Compare To Constant6 : simulink/Logic and Bit Operations/Compare To Constant  relop===  const=6  OutDataTypeStr=boolean
  Demux1 : Demux  Outputs=8
  Gain : Gain  OutDataTypeStr=uint8
  Gain1 : Gain  Gain=2  OutDataTypeStr=uint8
  Gain3 : Gain  Gain=4  OutDataTypeStr=uint8
  Integer to Bit Converter : commutil2/Integer to Bit Converter  nbits=8  signedInputValues=Unsigned  bitOrder=MSB first  outDtype=Inherit via internal rule
      settings: SourceProductBaseCode=SL
  Mux : Mux  Inputs=6
  Mux1 : Mux  Inputs=3
  OR : Logic  Operator=OR  Inputs=1  IconShape=distinctive  AllPortsSameDT=off  OutDataTypeStr=boolean
  Terminator : Terminator
  Abort : Outport
  Reset : Outport  Port=2
  Toggle : Outport  Port=3
  Error SCS : Outport  Port=4
  Segmented Response : Outport  Port=5
  wires:
  Compare To Constant3/1 -> Abort/1, Mux/4
  Domain Info/1 -> Integer to Bit Converter/1
  Integer to Bit Converter/1 -> Demux1/1
  Demux1/4 -> Toggle/1
  Demux1/8 -> Reset/1
  Demux1/1 -> Gain3/1
  Demux1/2 -> Gain1/1
  Gain1/1 -> Add2/2
  Gain3/1 -> Add2/1
  Gain/1 -> Add2/3
  Demux1/3 -> Gain/1
  Compare To Constant/1 -> Mux/1
  Add2/1 -> Compare To Constant4/1, Compare To Constant6/1, Compare To Constant3/1, Compare To Constant1/1, Compare To Constant5/1, Compare To Constant/1, Compare To Constant2/1
  Compare To Constant1/1 -> Mux/2
  Compare To Constant2/1 -> Mux/3
  Compare To Constant4/1 -> Mux/5
  Compare To Constant6/1 -> Mux/6
  Mux/1 -> OR/1
  OR/1 -> Error SCS/1
  Demux1/6 -> Mux1/2
  Demux1/5 -> Mux1/1
  Demux1/7 -> Mux1/3
  Mux1/1 -> Terminator/1
  Compare To Constant5/1 -> Segmented Response/1

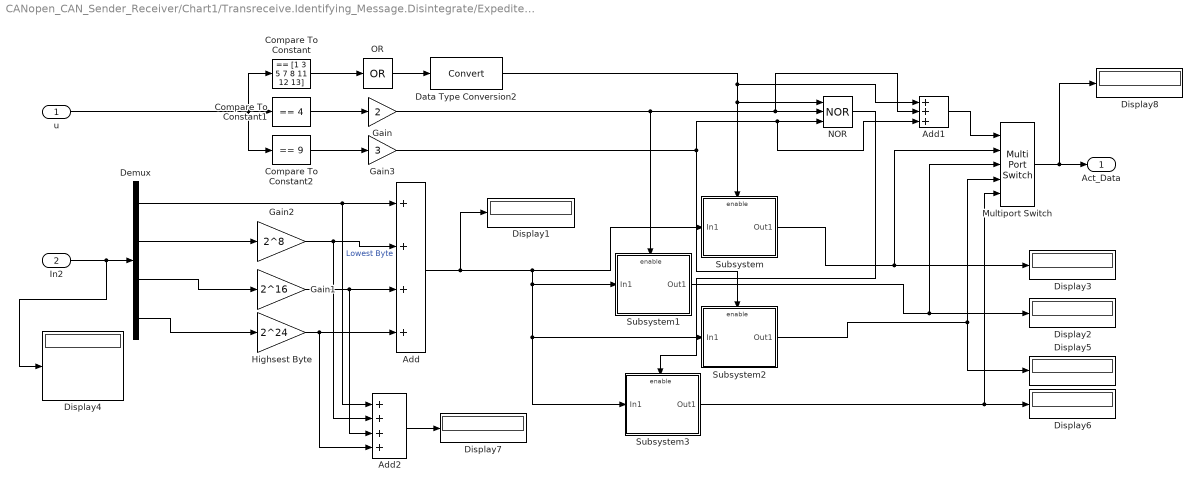
== system CANopen_CAN_Sender_Receiver/Chart1/Transreceive.Identifying_Message.Disintegrate/Expedite/Data Processing/Subsystem4 ==
  u : Inport
  In2 : Inport  Port=2
  Add : Sum  Inputs=++++
  Add1 : Sum  Inputs=+++
  Add2 : Sum  Inputs=++++
  Compare To Constant : simulink/Logic and Bit Operations/Compare To Constant  relop===  const=[1 3 5 7 8 11 12 13]  OutDataTypeStr=boolean
  Compare To Constant1 : simulink/Logic and Bit Operations/Compare To Constant  relop===  const=4  OutDataTypeStr=boolean
  Compare To Constant2 : simulink/Logic and Bit Operations/Compare To Constant  relop===  const=9  OutDataTypeStr=boolean
  Data Type Conversion2 : DataTypeConversion
  Demux : Demux
  Display{1..8} (8 alike) : Display
  Gain : Gain  Gain=2
  Gain1 : Gain  Gain=2^16
  Gain2 : Gain  Gain=2^8
  Gain3 : Gain  Gain=3
  Highsest Byte : Gain  Gain=2^24
  Multiport Switch : MultiPortSwitch  Inputs=4  DiagnosticForDefault=None  OutDataTypeStr=double
  NOR : Logic  Operator=NOR  Inputs=3  IconShape=distinctive  AllPortsSameDT=off  OutDataTypeStr=boolean
  OR : Logic  Operator=OR  Inputs=1  IconShape=distinctive  AllPortsSameDT=off  OutDataTypeStr=boolean
  Subsystem : Subsystem
  Subsystem1 : Subsystem
  Subsystem2 : Subsystem
  Subsystem3 : Subsystem
  Act_Data : Outport
  wires:
  Multiport Switch/1 -> Act_Data/1, Display8/1
  Gain2/1 -> Add/2, Add2/2
  Demux/3 -> Gain1/1
  Demux/4 -> Highsest Byte/1
  Demux/2 -> Gain2/1
  Subsystem1/1(Out1) -> Display2/1, Multiport Switch/3
  Add2/1 -> Display7/1
  u/1 -> Compare To Constant1/1, Compare To Constant/1, Compare To Constant2/1
  Data Type Conversion2/1 -> Subsystem/Enable, NOR/1, Add1/1
  Gain1/1 -> Add2/3, Add/3
  NOR/1 -> Subsystem3/Enable
  Subsystem3/1(Out1) -> Display6/1, Multiport Switch/5
  Demux/1 -> Add2/1, Add/1  "Lowest Byte"
  Subsystem/1(Out1) -> Display3/1, Multiport Switch/2
  Gain3/1 -> NOR/3, Add1/3, Subsystem2/Enable
  Subsystem2/1(Out1) -> Display5/1, Multiport Switch/4
  In2/1 -> Demux/1, Display4/1
  Compare To Constant/1 -> OR/1
  OR/1 -> Data Type Conversion2/1
  Add/1 -> Subsystem1/1(In1), Subsystem3/1(In1), Subsystem2/1(In1), Subsystem/1(In1), Display1/1
  Add1/1 -> Multiport Switch/1
  Compare To Constant1/1 -> Gain/1
  Highsest Byte/1 -> Add/4, Add2/4
  Compare To Constant2/1 -> Gain3/1
  Gain/1 -> NOR/2, Add1/2, Subsystem1/Enable

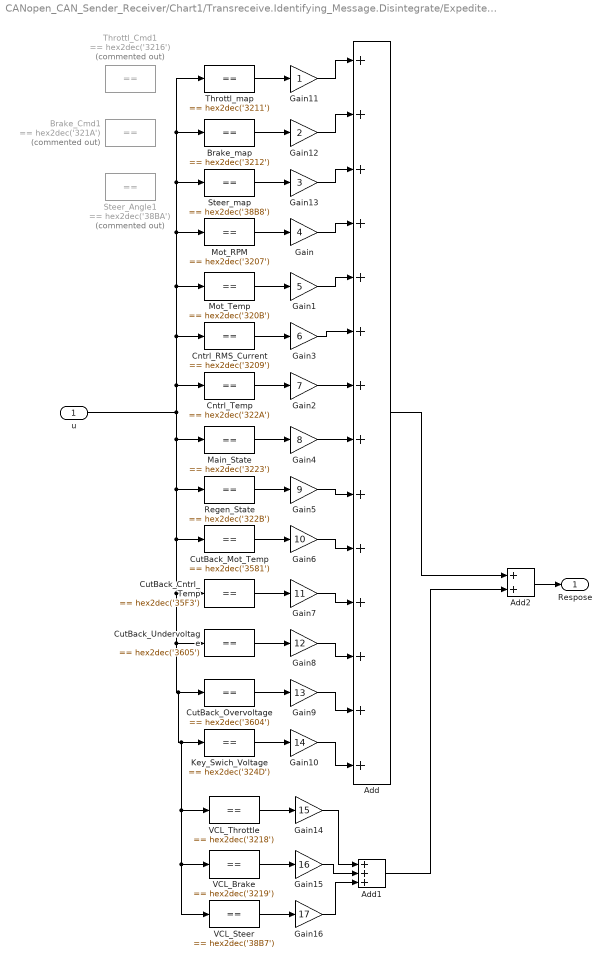
== system CANopen_CAN_Sender_Receiver/Chart1/Transreceive.Identifying_Message.Disintegrate/Expedite/MessageNumber/Read Messages ==
  u : Inport
  Add : Sum  Inputs=++++++++++++++
  Add1 : Sum  Inputs=+++
  Add2 : Sum
  Brake_Cmd1 : simulink/Logic and Bit Operations/Compare To Constant  Commented=on  relop===  const=hex2dec('321A')  OutDataTypeStr=uint8
  Brake_map : simulink/Logic and Bit Operations/Compare To Constant  relop===  const=hex2dec('3212')  OutDataTypeStr=uint8
  Cntrl_RMS_Current : simulink/Logic and Bit Operations/Compare To Constant  relop===  const=hex2dec('3209')  OutDataTypeStr=uint8
  Cntrl_Temp : simulink/Logic and Bit Operations/Compare To Constant  relop===  const=hex2dec('322A')  OutDataTypeStr=uint8
  CutBack_Cntrl_Temp : simulink/Logic and Bit Operations/Compare To Constant  relop===  const=hex2dec('35F3')  OutDataTypeStr=uint8
  CutBack_Mot_Temp : simulink/Logic and Bit Operations/Compare To Constant  relop===  const=hex2dec('3581')  OutDataTypeStr=uint8
  CutBack_Overvoltage : simulink/Logic and Bit Operations/Compare To Constant  relop===  const=hex2dec('3604')  OutDataTypeStr=uint8
  CutBack_Undervoltage : simulink/Logic and Bit Operations/Compare To Constant  relop===  const=hex2dec('3605')  OutDataTypeStr=uint8
  Gain : Gain  Gain=4
  Gain1 : Gain  Gain=5
  Gain10 : Gain  Gain=14
  Gain11 : Gain
  Gain12 : Gain  Gain=2
  Gain13 : Gain  Gain=3
  Gain14 : Gain  Gain=15
  Gain15 : Gain  Gain=16
  Gain16 : Gain  Gain=17
  Gain2 : Gain  Gain=7
  Gain3 : Gain  Gain=6
  Gain4 : Gain  Gain=8
  Gain5 : Gain  Gain=9
  Gain6 : Gain  Gain=10
  Gain7 : Gain  Gain=11
  Gain8 : Gain  Gain=12
  Gain9 : Gain  Gain=13
  Key_Swich_Voltage : simulink/Logic and Bit Operations/Compare To Constant  relop===  const=hex2dec('324D')  OutDataTypeStr=uint8
  Main_State : simulink/Logic and Bit Operations/Compare To Constant  relop===  const=hex2dec('3223')  OutDataTypeStr=uint8
  Mot_RPM : simulink/Logic and Bit Operations/Compare To Constant  relop===  const=hex2dec('3207')  OutDataTypeStr=uint8
  Mot_Temp : simulink/Logic and Bit Operations/Compare To Constant  relop===  const=hex2dec('320B')  OutDataTypeStr=uint8
  Regen_State : simulink/Logic and Bit Operations/Compare To Constant  relop===  const=hex2dec('322B')  OutDataTypeStr=uint8
  Steer_Angle1 : simulink/Logic and Bit Operations/Compare To Constant  Commented=on  relop===  const=hex2dec('38BA')  OutDataTypeStr=uint8
  Steer_map : simulink/Logic and Bit Operations/Compare To Constant  relop===  const=hex2dec('38B8')  OutDataTypeStr=uint8
  Throttl_Cmd1 : simulink/Logic and Bit Operations/Compare To Constant  Commented=on  relop===  const=hex2dec('3216')  OutDataTypeStr=uint8
  Throttl_map : simulink/Logic and Bit Operations/Compare To Constant  relop===  const=hex2dec('3211')  OutDataTypeStr=uint8
  VCL_Brake : simulink/Logic and Bit Operations/Compare To Constant  relop===  const=hex2dec('3219')  OutDataTypeStr=uint8
  VCL_Steer : simulink/Logic and Bit Operations/Compare To Constant  relop===  const=hex2dec('38B7')  OutDataTypeStr=uint8
  VCL_Throttle : simulink/Logic and Bit Operations/Compare To Constant  relop===  const=hex2dec('3218')  OutDataTypeStr=uint8
  Respose : Outport
  wires:
  Add2/1 -> Respose/1
  Gain14/1 -> Add1/1
  Gain16/1 -> Add1/3
  Gain15/1 -> Add1/2
  VCL_Throttle/1 -> Gain14/1
  VCL_Steer/1 -> Gain16/1
  Add1/1 -> Add2/2
  u/1 -> Key_Swich_Voltage/1, VCL_Throttle/1, VCL_Steer/1, VCL_Brake/1, CutBack_Overvoltage/1, CutBack_Undervoltage/1, CutBack_Cntrl_Temp/1, CutBack_Mot_Temp/1, Regen_State/1, Main_State/1, Mot_Temp/1, Mot_RPM/1, Brake_map/1, Throttl_map/1, Steer_map/1, Cntrl_RMS_Current/1, Cntrl_Temp/1
  VCL_Brake/1 -> Gain15/1
  Mot_Temp/1 -> Gain1/1
  Mot_RPM/1 -> Gain/1
  Cntrl_RMS_Current/1 -> Gain3/1
  Regen_State/1 -> Gain5/1
  Cntrl_Temp/1 -> Gain2/1
  Main_State/1 -> Gain4/1
  CutBack_Cntrl_Temp/1 -> Gain7/1
  CutBack_Mot_Temp/1 -> Gain6/1
  CutBack_Undervoltage/1 -> Gain8/1
  CutBack_Overvoltage/1 -> Gain9/1
  Key_Swich_Voltage/1 -> Gain10/1
  Steer_map/1 -> Gain13/1
  Brake_map/1 -> Gain12/1
  Throttl_map/1 -> Gain11/1
  Gain11/1 -> Add/1
  Gain12/1 -> Add/2
  Gain13/1 -> Add/3
  Gain/1 -> Add/4
  Gain1/1 -> Add/5
  Gain3/1 -> Add/6
  Gain2/1 -> Add/7
  Gain4/1 -> Add/8
  Gain5/1 -> Add/9
  Gain6/1 -> Add/10
  Gain7/1 -> Add/11
  Gain8/1 -> Add/12
  Gain9/1 -> Add/13
  Gain10/1 -> Add/14
  Add/1 -> Add2/1

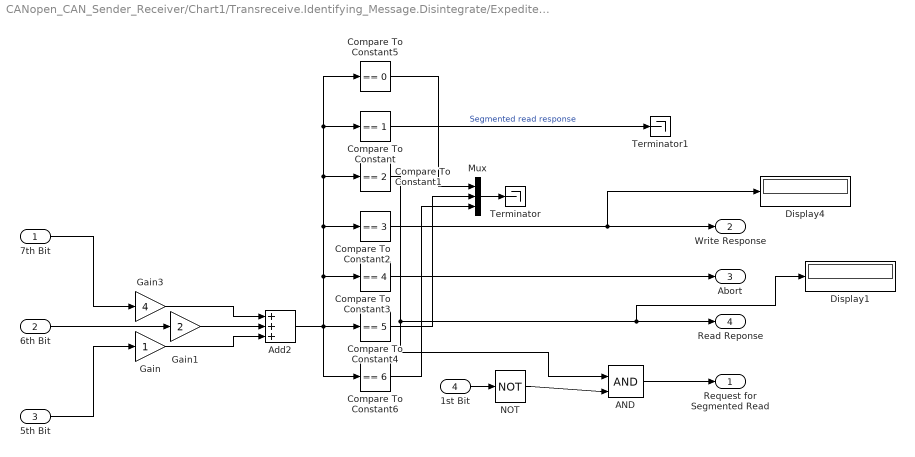
== system CANopen_CAN_Sender_Receiver/Chart1/Transreceive.Identifying_Message.Disintegrate/Expedite/MessageNumber/Subsystem ==
  7th Bit : Inport
  6th Bit : Inport  Port=2
  5th Bit : Inport  Port=3
  1st Bit : Inport  Port=4
  AND : Logic  IconShape=distinctive  AllPortsSameDT=off  OutDataTypeStr=boolean
  Add2 : Sum  Inputs=+++
  Compare To Constant : simulink/Logic and Bit Operations/Compare To Constant  relop===  const=1  OutDataTypeStr=boolean
  Compare To Constant1 : simulink/Logic and Bit Operations/Compare To Constant  relop===  const=2  OutDataTypeStr=boolean
  Compare To Constant2 : simulink/Logic and Bit Operations/Compare To Constant  relop===  const=3  OutDataTypeStr=boolean
  Compare To Constant3 : simulink/Logic and Bit Operations/Compare To Constant  relop===  const=4  OutDataTypeStr=boolean
  Compare To Constant4 : simulink/Logic and Bit Operations/Compare To Constant  relop===  const=5  OutDataTypeStr=boolean
  Compare To Constant5 : simulink/Logic and Bit Operations/Compare To Constant  relop===  const=0  OutDataTypeStr=boolean
  Compare To Constant6 : simulink/Logic and Bit Operations/Compare To Constant  relop===  const=6  OutDataTypeStr=boolean
  Display1 : Display
  Display4 : Display
  Gain : Gain
  Gain1 : Gain  Gain=2
  Gain3 : Gain  Gain=4
  Mux : Mux  Inputs=3
  NOT : Logic  Operator=NOT  IconShape=distinctive  AllPortsSameDT=off  OutDataTypeStr=boolean
  Terminator : Terminator
  Terminator1 : Terminator
  "Request for Segmented Read " : Outport
  Write Response : Outport  Port=2
  Abort : Outport  Port=3
  Read Reponse : Outport  Port=4
  wires:
  Compare To Constant5/1 -> Mux/1
  Compare To Constant4/1 -> Mux/2
  Add2/1 -> Compare To Constant3/1, Compare To Constant1/1, Compare To Constant5/1, Compare To Constant/1, Compare To Constant2/1, Compare To Constant4/1, Compare To Constant6/1
  Compare To Constant/1 -> Terminator1/1  "Segmented read response"
  1st Bit/1 -> NOT/1
  Mux/1 -> Terminator/1
  5th Bit/1 -> Gain/1
  NOT/1 -> AND/2
  Compare To Constant6/1 -> Mux/3
  Gain/1 -> Add2/3
  Gain3/1 -> Add2/1
  Gain1/1 -> Add2/2
  Compare To Constant3/1 -> Abort/1
  AND/1 -> "Request for Segmented Read "/1
  Compare To Constant2/1 -> Write Response/1, Display4/1
  6th Bit/1 -> Gain1/1
  7th Bit/1 -> Gain3/1
  Compare To Constant1/1 -> Read Reponse/1, Display1/1, AND/1

== system CANopen_CAN_Sender_Receiver/Chart1/Transreceive.Identifying_Message.Disintegrate/Expedite/Data Processing/Subsystem4/Subsystem ==
  In1 : Inport
  Enable : EnablePort  StatesWhenEnabling=reset
  Data Type Conversion : DataTypeConversion  OutDataTypeStr=int16  SaturateOnIntegerOverflow=on
  Out1 : Outport
  wires:
  Data Type Conversion/1 -> Out1/1
  In1/1 -> Data Type Conversion/1

== system CANopen_CAN_Sender_Receiver/Chart1/Transreceive.Identifying_Message.Disintegrate/Expedite/Data Processing/Subsystem4/Subsystem1 ==
  In1 : Inport
  Enable : EnablePort  StatesWhenEnabling=reset
  Data Type Conversion1 : DataTypeConversion  OutDataTypeStr=int32  SaturateOnIntegerOverflow=on
  Out1 : Outport
  wires:
  Data Type Conversion1/1 -> Out1/1
  In1/1 -> Data Type Conversion1/1

== system CANopen_CAN_Sender_Receiver/Chart1/Transreceive.Identifying_Message.Disintegrate/Expedite/Data Processing/Subsystem4/Subsystem2 ==
  In1 : Inport
  Enable : EnablePort  StatesWhenEnabling=reset
  Data Type Conversion4 : DataTypeConversion  OutDataTypeStr=uint8  SaturateOnIntegerOverflow=on
  Out1 : Outport
  wires:
  In1/1 -> Data Type Conversion4/1
  Data Type Conversion4/1 -> Out1/1

== system CANopen_CAN_Sender_Receiver/Chart1/Transreceive.Identifying_Message.Disintegrate/Expedite/Data Processing/Subsystem4/Subsystem3 ==
  In1 : Inport
  Enable : EnablePort  StatesWhenEnabling=reset
  Data Type Conversion3 : DataTypeConversion  OutDataTypeStr=uint16  SaturateOnIntegerOverflow=on
  Out1 : Outport
  wires:
  In1/1 -> Data Type Conversion3/1
  Data Type Conversion3/1 -> Out1/1
